simulink model "mdl_filterung"  (Simulink 8.6)
settings: Solver=FixedStepDiscrete  StartTime=0.0  StopTime=t_end  FixedStep=t_sample  RelTol=1e-3
PostLoadFcn:
  | , if any(exist('dsrtsu_mdlpostloadfcn', 'file') == [2, 3, 6]), try dsrtsu_mdlpostloadfcn('Execute', bdroot); catch fprintf('Error in PostLoadFcn (dsrtsu_mdlpostloadfcn) for model "%s":\n %s\n', bdroot, lasterr); end, end,
undefined symbols (not defined in the file): t_sample
settings Model: DSRTSU_INTERNAL_RTI_VER=360  DSRTSU_INTERNAL_RTI_TYPE=rti1103  Creator=Schaper  LastModifiedBy=Amann
settings OptimizationCC: BlockReduction=off  OptimizeBlockIOStorage=off  BufferReuse=off  GlobalBufferReuse=off  ExpressionFolding=off  LocalBlockOutputs=off
settings DebuggingCC: FcnCallInpInsideContextMsg=UseLocalSettings
settings HardwareCC: ProdIntDivRoundTo=Zero  ProdEndianess=BigEndian  ProdHWDeviceType=Generic->Custom  TargetIntDivRoundTo=Zero  TargetEndianess=BigEndian  TargetHWDeviceType=Generic->Custom
settings RTWCC: SystemTargetFile=rti1103.tlc  MakeCommand=make_rti  TemplateMakefile=rti1103.tmf  Description=dSPACE DS1103 Hardware Platform
settings STFCustomTargetCC: ParMdlRefBuildCompliant=on  GeneratePreprocessorConditionals=Disable all  MatFileLogging=on  CPPClassGenCompliant=on  SystemTargetFile=rti1103.tlc
settings GRTTargetCC: CompOptLevelCompliant=off  ConcurrentExecutionCompliant=off  UseToolchainInfoCompliant=off  ExtModeMexFile=noextcomm
settings CustomProperty: DataType=RTWOptions_EnumType_C__Programme_dSPACE66_matlab_rti1103_tlc_rti1103_1InitialSimState  Value=RUN
settings EnumStrPairs: String=RUN

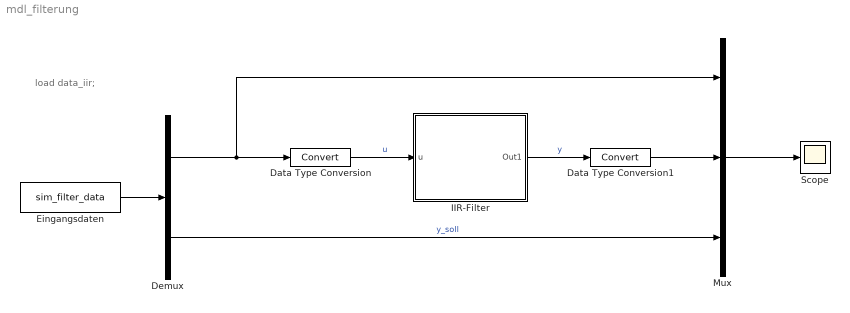
== system mdl_filterung ==
  note: load data_iir;
  Data Type Conversion : DataTypeConversion
  Data Type Conversion1 : DataTypeConversion
  Demux : Demux  Outputs=2
  Eingangsdaten : FromWorkspace  VariableName=sim_filter_data  SampleTime=t_sample
  IIR-Filter : Subsystem  mask{b=0, a=0}
      mask prompts: b "Zähler-Koeffizienten b"; a "Nenner-Koeffizienten a"
  Mux : Mux  Inputs=3
  Scope : Scope
  wires:
  Mux/1 -> Scope/1
  Data Type Conversion/1 -> IIR-Filter/1(u)  "u"
  IIR-Filter/1(Out1) -> Data Type Conversion1/1  "y"
  Eingangsdaten/1 -> Demux/1
  Demux/1 -> Mux/1, Data Type Conversion/1
  Demux/2 -> Mux/3  "y_soll"
  Data Type Conversion1/1 -> Mux/2

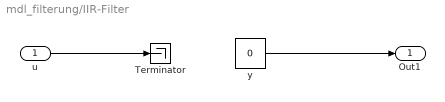
== system mdl_filterung/IIR-Filter ==
  u : Inport
  Terminator : Terminator
  y : Constant  Value=0
  Out1 : Outport
  wires:
  u/1 -> Terminator/1
  y/1 -> Out1/1
